simulink model "Battery"  (R2021b)
settings: Solver=VariableStepAuto  StartTime=0.0  StopTime=10.0  RelTol=1e-3
model workspace (MAT data in the model file):
  C = 7
  PD = 120
  S = 4
undefined symbols (not defined in the file or in its folder): Ion, Lithium
libraries: spsBatteryLib x1, spsControlledCurrentSourceLib x1, simulink x1, spspowerguiLib x1
settings Model: Creator=aakas  LastModifiedBy=aakas

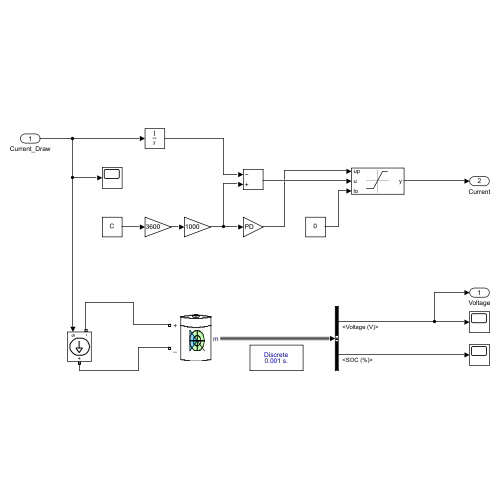
[thumbnail: Simulink's stored preview of the top-level diagram]
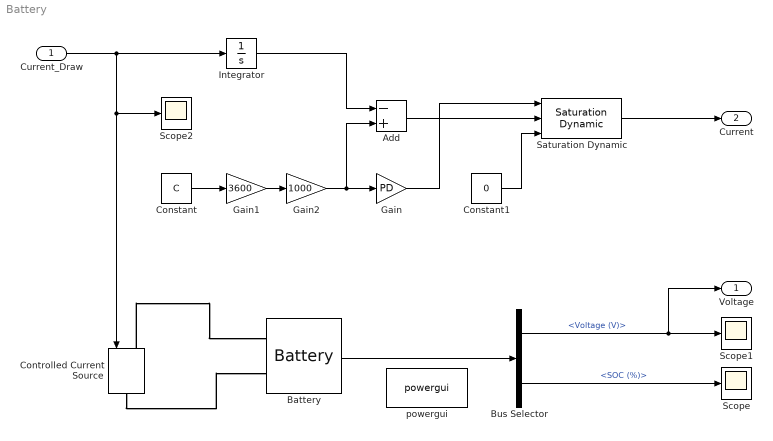
== system Battery ==
  Current_Draw : Inport
  Add : Sum  Inputs=-+
  Battery : spsBatteryLib/Battery  BatType=Lithium-Ion  ShowTempParam=off  ThermalPreset="11.1V  6600mAh  (LiCoO2)"  ShowAgeParam=off  NomV=3.7*S  NomQ=C  SOC=100  Batt_Tr=30  PresetModel=on  MaxQ=7000  MinV=11.1  FullV=17.227  Dis_rate=3043.4783  R=2.1143e-05  Normal_OP=6330.4348  expZone="[15.98971       343.913]"  current=[6.5 13 32.5]  Units=Time  Tci=20  NomT=20  T2=-30  MaxQ2=4.8  FullV2=7.1  Normal_OP2=5.655  expZone2="[6.58           1]"  Rca=0.6  ti=2000  Dp=0  Neq0=0  Tsim=1e6  Ta1=25  Qeol=5.4*0.9  Reol=0.013333*1.2  Char_age=[2.3478, 3]  Dis_age=[2.3478, 10]  N1=1500  N2=10500  N3=1000  N4=1400  Ta2=45  N5=950
  Bus Selector : BusSelector  OutputSignals=Voltage (V),SOC (%)
  Constant : Constant  Value=C  SampleTime=Inf
  Constant1 : Constant  Value=0
  Controlled Current Source : spsControlledCurrentSourceLib/Controlled Current Source  Initialize=on  Source_Type=AC  Amplitude=0  Phase=0  Frequency=0  Measurements=None
  Gain : Gain  Gain=PD
  Gain1 : Gain  Gain=3600
  Gain2 : Gain  Gain=1000
  Integrator : Integrator
  Saturation Dynamic : simulink/Discontinuities/Saturation Dynamic  OutMin=[]  OutMax=[]  OutDataTypeStr=Inherit: Same as second input  OutDataType=fixdt(1, 16)  OutScaling=2^-10  DoSatur=off
  Scope : Scope
  Scope1 : Scope
  Scope2 : Scope
  powergui : spspowerguiLib/powergui  Priority=1  SimulationMode=Discrete  SampleTime=0.001  frequency=60  Iterations=50  frequencyindice=0  Pbase=100e6  ErrMax=1e-4  UnitsV=kV  UnitsW=MW  buscounter=0  FunctionMessages=off  echomessages=off  EnableUseOfTLC=off  CurrentSourceSwitches=off  DisableSnubberDevices=off  DisableRonSwitches=off  DisableVfSwitches=off  DisplayEquations=off  AutomaticDiscreteSolvers=off  SolverType=Tustin/Backward Euler (TBE)  Interpol=off  ExternalGateDelay=off  methode=off  Ts=100  x0status=blocks  SPID=on  SwTol=0  HookPort=off  NonlinearTolerance=1e-4  nMaxIteration=100  ContinueOnMaxIteration=off  RestoreLinks=warning  ResistiveCurrentMeasurement=off  Frange=[0:2:500]  Ylog=off  Xlog=on  ShowGrid=off  save=off  variable=ZData  structure=0  ZoomFFT=off  StartTime=0.0  cycles=1  DisplayStyle=1  fundamental=60  FreqAxis=off  MaxFrequency=1000  frequencyindicesteady=1  RmsSteady=1  display=off
  Voltage : Outport
  Current : Outport  Port=2
  wires:
  Integrator/1 -> Add/1
  Gain2/1 -> Gain/1, Add/2
  Add/1 -> Saturation Dynamic/2
  Gain/1 -> Saturation Dynamic/1
  Constant1/1 -> Saturation Dynamic/3
  Saturation Dynamic/1 -> Current/1
  Battery/1 -> Bus Selector/1
  Bus Selector/1 -> Voltage/1, Scope1/1  "<Voltage (V)>"
  Bus Selector/2 -> Scope/1  "<SOC (%)>"
  Current_Draw/1 -> Scope2/1, Controlled Current Source/1, Integrator/1
  Constant/1 -> Gain1/1
  Gain1/1 -> Gain2/1
  connections:
  Controlled Current Source/RConn1 -- Battery/LConn2
  Controlled Current Source/LConn1 -- Battery/LConn1
